simulink model "gyro"  (R2020a)
settings: Solver=daessc  StartTime=0.0  StopTime=0.35  RelTol=1e-3
values from neighbouring files (symbols this model uses):
  m = 0.5    [init_2021_03_10.m]
  ts = 1e-4    (= 0.0001)    [init_2021_03_10.m]
libraries: fl_lib x33, nesl_utility x8
settings Model: Creator=dbagn  LastModifiedBy=dbagn

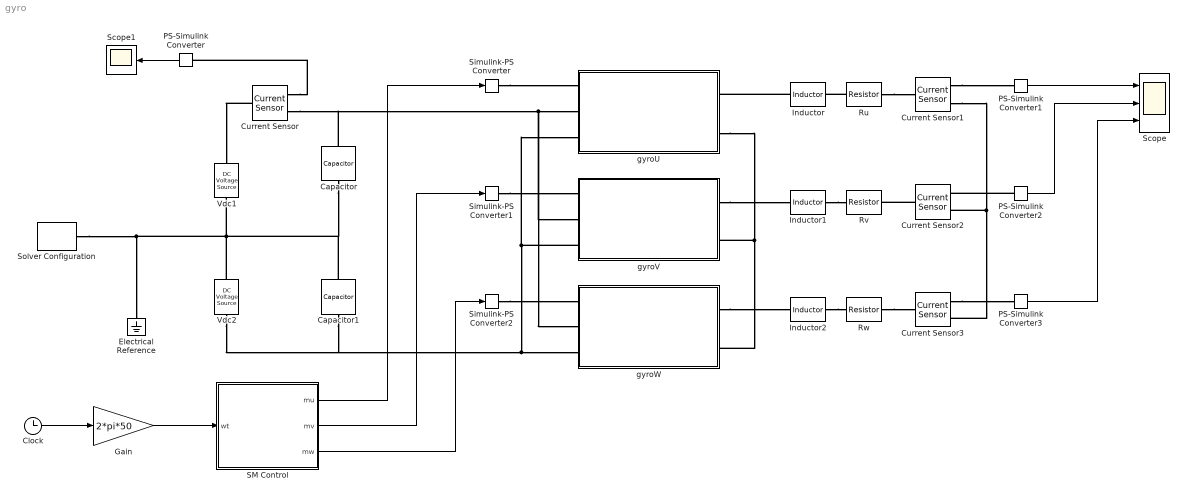
== system gyro ==
  Capacitor : fl_lib/Electrical/Electrical Elements/Capacitor  c=5e-3 F  r=1e-3 Ohm  g=0 1/Ohm  i_specify=off  i_priority=None  i=0 A  i_nominal_specify=off  i_nominal_unit=A  i_nominal_value=1  v_specify=off  v_priority=High  v=350 V  v_nominal_specify=off  v_nominal_unit=V  v_nominal_value=1  vc_specify=on  vc_priority=High  vc=350 V  vc_nominal_specify=off  vc_nominal_unit=V  vc_nominal_value=1
  Capacitor1 : fl_lib/Electrical/Electrical Elements/Capacitor  c=5e-3 F  r=1e-3 Ohm  g=0 1/Ohm  i_specify=off  i_priority=None  i=0 A  i_nominal_specify=off  i_nominal_unit=A  i_nominal_value=1  v_specify=off  v_priority=High  v=0 V  v_nominal_specify=off  v_nominal_unit=V  v_nominal_value=1  vc_specify=on  vc_priority=High  vc=350 V  vc_nominal_specify=off  vc_nominal_unit=V  vc_nominal_value=1
  Clock : Clock
  Current Sensor{,1..3} (4 alike) : fl_lib/Electrical/Electrical Sensors/Current Sensor
  Electrical Reference : fl_lib/Electrical/Electrical Elements/Electrical Reference
  Gain : Gain  Gain=2*pi*50
  Inductor : fl_lib/Electrical/Electrical Elements/Inductor  l=1e-4 H  r=0 Ohm  g=1e-9 1/Ohm  i_specify=off  i_priority=None  i=0 A  i_nominal_specify=off  i_nominal_unit=A  i_nominal_value=1  v_specify=off  v_priority=None  v=0 V  v_nominal_specify=off  v_nominal_unit=V  v_nominal_value=1  i_L_specify=off  i_L_priority=High  i_L=0 A  i_L_nominal_specify=off  i_L_nominal_unit=A  i_L_nominal_value=1
  Inductor1 : fl_lib/Electrical/Electrical Elements/Inductor  l=1e-4 H  r=0 Ohm  g=1e-9 1/Ohm  i_specify=off  i_priority=None  i=0 A  i_nominal_specify=off  i_nominal_unit=A  i_nominal_value=1  v_specify=off  v_priority=None  v=0 V  v_nominal_specify=off  v_nominal_unit=V  v_nominal_value=1  i_L_specify=off  i_L_priority=High  i_L=0 A  i_L_nominal_specify=off  i_L_nominal_unit=A  i_L_nominal_value=1
  Inductor2 : fl_lib/Electrical/Electrical Elements/Inductor  l=1e-4 H  r=0 Ohm  g=1e-9 1/Ohm  i_specify=off  i_priority=None  i=0 A  i_nominal_specify=off  i_nominal_unit=A  i_nominal_value=1  v_specify=off  v_priority=None  v=0 V  v_nominal_specify=off  v_nominal_unit=V  v_nominal_value=1  i_L_specify=off  i_L_priority=High  i_L=0 A  i_L_nominal_specify=off  i_L_nominal_unit=A  i_L_nominal_value=1
  PS-Simulink Converter{,1..3} (4 alike) : nesl_utility/PS-Simulink Converter  PhysicalDomain=network_engine_domain  SubClassName=ps_output  LeftPortType=input  RightPortType=output  PseudoPeriodic=off  Frequencies=[]  Unit=inherit  AffineConversion=off
  Ru : fl_lib/Electrical/Electrical Elements/Resistor  R=20 Ohm  i_specify=off  i_priority=None  i=0 A  i_nominal_specify=off  i_nominal_unit=A  i_nominal_value=1  v_specify=off  v_priority=None  v=0 V  v_nominal_specify=off  v_nominal_unit=V  v_nominal_value=1
  Rv : fl_lib/Electrical/Electrical Elements/Resistor  R=20 Ohm  i_specify=off  i_priority=None  i=0 A  i_nominal_specify=off  i_nominal_unit=A  i_nominal_value=1  v_specify=off  v_priority=None  v=0 V  v_nominal_specify=off  v_nominal_unit=V  v_nominal_value=1
  Rw : fl_lib/Electrical/Electrical Elements/Resistor  R=20 Ohm  i_specify=off  i_priority=None  i=0 A  i_nominal_specify=off  i_nominal_unit=A  i_nominal_value=1  v_specify=off  v_priority=None  v=0 V  v_nominal_specify=off  v_nominal_unit=V  v_nominal_value=1
  SM Control : Subsystem
  Scope : Scope  NumInputPorts=3
  Scope1 : Scope
  Simulink-PS Converter : nesl_utility/Simulink-PS Converter  PhysicalDomain=network_engine_domain  SubClassName=ps_input  LeftPortType=input  RightPortType=output  PseudoPeriodic=off  Frequencies=[]  NoiseDistribution=none  NoiseParameters=[]  Unit=1  AffineConversion=off  FilteringAndDerivatives=provide  SimscapeFilterOrder=1  InputFilterTimeConstant=0.001  UdotUserProvided=0
  Simulink-PS Converter1 : nesl_utility/Simulink-PS Converter  PhysicalDomain=network_engine_domain  SubClassName=ps_input  LeftPortType=input  RightPortType=output  PseudoPeriodic=off  Frequencies=[]  NoiseDistribution=none  NoiseParameters=[]  Unit=1  AffineConversion=off  FilteringAndDerivatives=provide  SimscapeFilterOrder=1  InputFilterTimeConstant=0.001  UdotUserProvided=0
  Simulink-PS Converter2 : nesl_utility/Simulink-PS Converter  PhysicalDomain=network_engine_domain  SubClassName=ps_input  LeftPortType=input  RightPortType=output  PseudoPeriodic=off  Frequencies=[]  NoiseDistribution=none  NoiseParameters=[]  Unit=1  AffineConversion=off  FilteringAndDerivatives=provide  SimscapeFilterOrder=1  InputFilterTimeConstant=0.001  UdotUserProvided=0
  Solver Configuration : nesl_utility/Solver Configuration  PhysicalDomain=network_engine_domain  SubClassName=solver  LeftPortType=input  RightPortType=generic  Tones=[]  Harmonics=[]  SimulateNoise=off  Profile=off  UseLocalSampling=off  EnableSwitchedLinearOptims=on  FrequencyDomain=off  UseCCode=off  RelTol=0.001  AbsTol=1e-06  MinStep=1e-09  ToWorkspace=off  RevertToSquareIcSolve=off  NumHomotopyIterations=100  PhasorMode=off  PhasorModeNumHarmonics=1  DoDC=off  ResidualTolerance=1e-09  UseLocalSolver=on  LocalSolverChoice=NE_BACKWARD_EULER_ADVANCER  LocalSolverSampleTime=ts  DoFixedCost=on  MaxNonlinIter=3  MaxModeIter=2  LinearAlgebra=auto  EquationFormulation=NE_TIME_EF  DelaysMemoryBudget=1024  AutomaticFiltering=on  FilteringTimeConstant=0.001  PartitionStorageMethod=AS_NEEDED  PartitionMemoryBudget=1024  PartitionMethod=ROBUST
  Vdc1 : fl_lib/Electrical/Electrical Sources/DC Voltage Source  v0=350 V
  Vdc2 : fl_lib/Electrical/Electrical Sources/DC Voltage Source  v0=350 V
  gyroU : Subsystem
  gyroV : Subsystem
  gyroW : Subsystem
  wires:
  Clock/1 -> Gain/1
  Gain/1 -> SM Control/1(wt)
  SM Control/1(mu) -> Simulink-PS Converter/1
  SM Control/2(mv) -> Simulink-PS Converter1/1
  SM Control/3(mw) -> Simulink-PS Converter2/1
  PS-Simulink Converter1/1 -> Scope/1
  PS-Simulink Converter2/1 -> Scope/2
  PS-Simulink Converter3/1 -> Scope/3
  PS-Simulink Converter/1 -> Scope1/1
  connections:
  gyroW/LConn2 -- gyroV/LConn2 -- Capacitor/LConn1 -- Current Sensor/RConn2 -- gyroU/LConn2
  Vdc2/LConn1 -- Capacitor1/LConn1 -- Capacitor/RConn1 -- Solver Configuration/RConn1 -- Electrical Reference/LConn1 -- Vdc1/RConn1
  gyroV/LConn3 -- Capacitor1/RConn1 -- Vdc2/RConn1 -- gyroW/LConn3 -- gyroU/LConn3
  gyroU/RConn2 -- gyroW/RConn2 -- gyroV/RConn2
  Ru/LConn1 -- Inductor/RConn1
  Inductor1/RConn1 -- Rv/LConn1
  gyroW/RConn1 -- Inductor2/LConn1
  Simulink-PS Converter/RConn1 -- gyroU/LConn1
  Simulink-PS Converter1/RConn1 -- gyroV/LConn1
  Simulink-PS Converter2/RConn1 -- gyroW/LConn1
  Current Sensor/LConn1 -- Vdc1/LConn1
  Current Sensor/RConn1 -- PS-Simulink Converter/LConn1
  Ru/RConn1 -- Current Sensor1/LConn1
  Current Sensor2/LConn1 -- Rv/RConn1
  Rw/RConn1 -- Current Sensor3/LConn1
  Current Sensor1/RConn2 -- Current Sensor3/RConn2 -- Current Sensor2/RConn2
  Current Sensor1/RConn1 -- PS-Simulink Converter1/LConn1
  PS-Simulink Converter2/LConn1 -- Current Sensor2/RConn1
  Current Sensor3/RConn1 -- PS-Simulink Converter3/LConn1
  Inductor/LConn1 -- gyroU/RConn1
  gyroV/RConn1 -- Inductor1/LConn1
  Inductor2/RConn1 -- Rw/LConn1

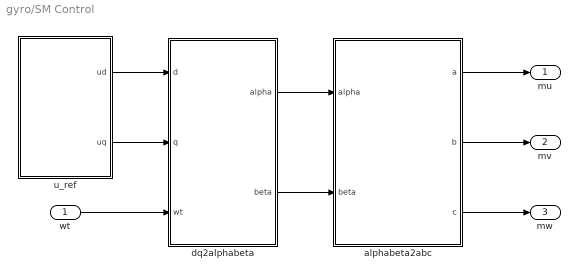
== system gyro/SM Control ==
  wt : Inport
  alphabeta2abc : Subsystem
  dq2alphabeta : Subsystem
  u_ref : Subsystem
  mu : Outport  VectorParamsAs1DForOutWhenUnconnected=off
  mv : Outport  Port=2  VectorParamsAs1DForOutWhenUnconnected=off
  mw : Outport  Port=3  VectorParamsAs1DForOutWhenUnconnected=off
  wires:
  wt/1 -> dq2alphabeta/3(wt)
  u_ref/2(uq) -> dq2alphabeta/2(q)
  u_ref/1(ud) -> dq2alphabeta/1(d)
  dq2alphabeta/2(beta) -> alphabeta2abc/2(beta)
  dq2alphabeta/1(alpha) -> alphabeta2abc/1(alpha)
  alphabeta2abc/1(a) -> mu/1
  alphabeta2abc/2(b) -> mv/1
  alphabeta2abc/3(c) -> mw/1

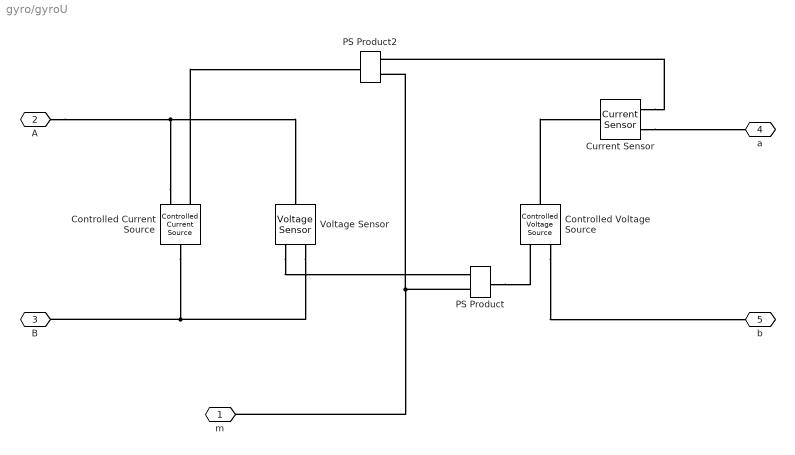
== system gyro/gyroU ==
  Controlled Current Source : fl_lib/Electrical/Electrical Sources/Controlled Current Source
  Controlled Voltage Source : fl_lib/Electrical/Electrical Sources/Controlled Voltage Source
  Current Sensor : fl_lib/Electrical/Electrical Sensors/Current Sensor
  PS Product : fl_lib/Physical Signals/Functions/PS Product
  PS Product2 : fl_lib/Physical Signals/Functions/PS Product
  Voltage Sensor : fl_lib/Electrical/Electrical Sensors/Voltage Sensor
  m : PMIOPort  Side=Left
  A : PMIOPort  Port=2  Side=Left
  B : PMIOPort  Port=3  Side=Left
  a : PMIOPort  Port=4  Side=Right
  b : PMIOPort  Port=5  Side=Right
  connections:
  Controlled Voltage Source/LConn1 -- Current Sensor/LConn1
  Controlled Voltage Source/RConn2 -- b/RConn1
  Controlled Current Source/RConn1 -- PS Product2/RConn1
  Controlled Current Source/RConn2 -- A/RConn1 -- Voltage Sensor/LConn1
  PS Product/LConn2 -- PS Product2/LConn1 -- m/RConn1
  Controlled Current Source/LConn1 -- B/RConn1 -- Voltage Sensor/RConn2
  Current Sensor/RConn2 -- a/RConn1
  PS Product/RConn1 -- Controlled Voltage Source/RConn1
  Voltage Sensor/RConn1 -- PS Product/LConn1
  Current Sensor/RConn1 -- PS Product2/LConn2

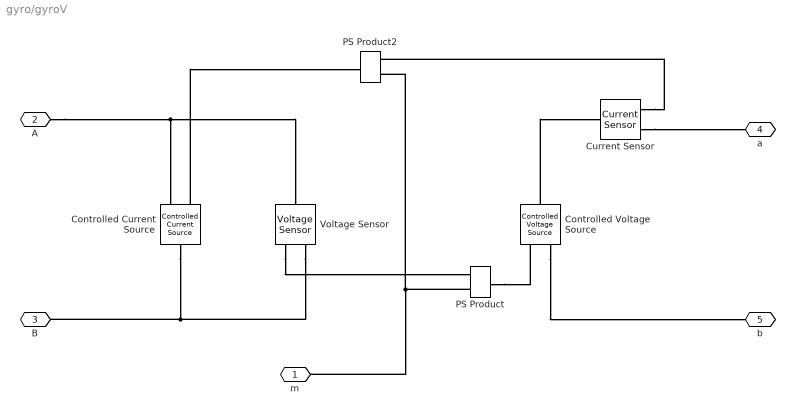
== system gyro/gyroV ==
  Controlled Current Source : fl_lib/Electrical/Electrical Sources/Controlled Current Source
  Controlled Voltage Source : fl_lib/Electrical/Electrical Sources/Controlled Voltage Source
  Current Sensor : fl_lib/Electrical/Electrical Sensors/Current Sensor
  PS Product : fl_lib/Physical Signals/Functions/PS Product
  PS Product2 : fl_lib/Physical Signals/Functions/PS Product
  Voltage Sensor : fl_lib/Electrical/Electrical Sensors/Voltage Sensor
  m : PMIOPort  Side=Left
  A : PMIOPort  Port=2  Side=Left
  B : PMIOPort  Port=3  Side=Left
  a : PMIOPort  Port=4  Side=Right
  b : PMIOPort  Port=5  Side=Right
  connections:
  Current Sensor/RConn1 -- PS Product2/LConn2
  Voltage Sensor/RConn1 -- PS Product/LConn1
  PS Product/RConn1 -- Controlled Voltage Source/RConn1
  Current Sensor/RConn2 -- a/RConn1
  B/RConn1 -- Controlled Current Source/LConn1 -- Voltage Sensor/RConn2
  PS Product2/LConn1 -- PS Product/LConn2 -- m/RConn1
  A/RConn1 -- Controlled Current Source/RConn2 -- Voltage Sensor/LConn1
  Controlled Current Source/RConn1 -- PS Product2/RConn1
  Controlled Voltage Source/RConn2 -- b/RConn1
  Controlled Voltage Source/LConn1 -- Current Sensor/LConn1

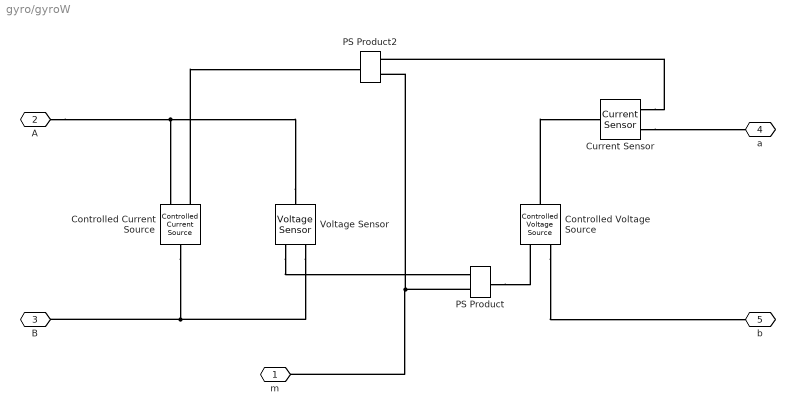
== system gyro/gyroW ==
  Controlled Current Source : fl_lib/Electrical/Electrical Sources/Controlled Current Source
  Controlled Voltage Source : fl_lib/Electrical/Electrical Sources/Controlled Voltage Source
  Current Sensor : fl_lib/Electrical/Electrical Sensors/Current Sensor
  PS Product : fl_lib/Physical Signals/Functions/PS Product
  PS Product2 : fl_lib/Physical Signals/Functions/PS Product
  Voltage Sensor : fl_lib/Electrical/Electrical Sensors/Voltage Sensor
  m : PMIOPort  Side=Left
  A : PMIOPort  Port=2  Side=Left
  B : PMIOPort  Port=3  Side=Left
  a : PMIOPort  Port=4  Side=Right
  b : PMIOPort  Port=5  Side=Right
  connections:
  Controlled Voltage Source/LConn1 -- Current Sensor/LConn1
  Controlled Voltage Source/RConn2 -- b/RConn1
  Controlled Current Source/RConn1 -- PS Product2/RConn1
  Voltage Sensor/LConn1 -- Controlled Current Source/RConn2 -- A/RConn1
  m/RConn1 -- PS Product/LConn2 -- PS Product2/LConn1
  Voltage Sensor/RConn2 -- Controlled Current Source/LConn1 -- B/RConn1
  Current Sensor/RConn2 -- a/RConn1
  PS Product/RConn1 -- Controlled Voltage Source/RConn1
  Voltage Sensor/RConn1 -- PS Product/LConn1
  Current Sensor/RConn1 -- PS Product2/LConn2

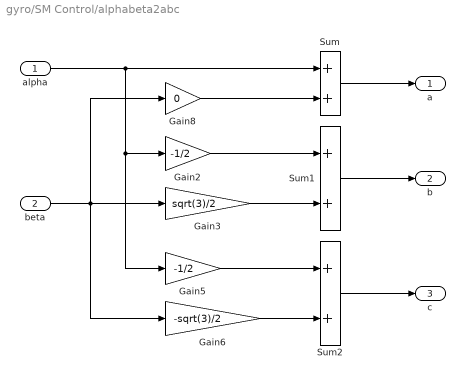
== system gyro/SM Control/alphabeta2abc ==
  alpha : Inport
  beta : Inport  Port=2
  Gain2 : Gain  Gain=-1/2
  Gain3 : Gain  Gain=sqrt(3)/2
  Gain5 : Gain  Gain=-1/2
  Gain6 : Gain  Gain=-sqrt(3)/2
  Gain8 : Gain  Gain=0
  Sum : Sum
  Sum1 : Sum
  Sum2 : Sum
  a : Outport  VectorParamsAs1DForOutWhenUnconnected=off
  b : Outport  Port=2  VectorParamsAs1DForOutWhenUnconnected=off
  c : Outport  Port=3  VectorParamsAs1DForOutWhenUnconnected=off
  wires:
  Gain2/1 -> Sum1/1
  Gain3/1 -> Sum1/2
  Gain5/1 -> Sum2/1
  Gain6/1 -> Sum2/2
  alpha/1 -> Sum/1, Gain2/1, Gain5/1
  beta/1 -> Gain3/1, Gain6/1, Gain8/1
  Sum/1 -> a/1
  Sum1/1 -> b/1
  Sum2/1 -> c/1
  Gain8/1 -> Sum/2

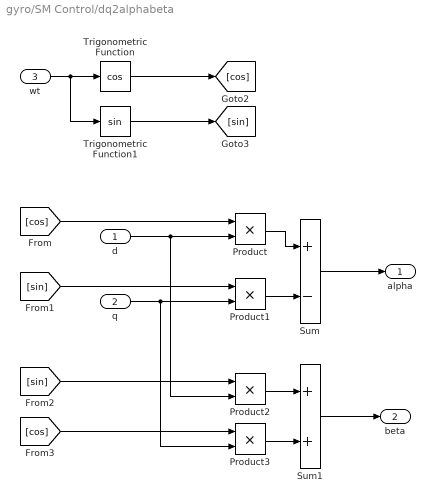
== system gyro/SM Control/dq2alphabeta ==
  d : Inport
  q : Inport  Port=2
  wt : Inport  Port=3
  Product{,1..3} (4 alike) : Product  RndMeth=Zero
  Sum : Sum  Inputs=+-
  Sum1 : Sum
  Trigonometric Function : Trigonometry  Operator=cos
  Trigonometric Function1 : Trigonometry
  alpha : Outport  VectorParamsAs1DForOutWhenUnconnected=off
  beta : Outport  Port=2  VectorParamsAs1DForOutWhenUnconnected=off
  wires:
  Sum1/1 -> beta/1
  [cos] -> Product3/1
  Product3/1 -> Sum1/2
  Product2/1 -> Sum1/1
  [sin] -> Product2/1
  Sum/1 -> alpha/1
  q/1 -> Product3/2, Product1/2
  [sin] -> Product1/1
  Product1/1 -> Sum/2
  Product/1 -> Sum/1
  d/1 -> Product2/2, Product/2
  [cos] -> Product/1
  Trigonometric Function1/1 -> [sin]
  Trigonometric Function/1 -> [cos]
  wt/1 -> Trigonometric Function/1, Trigonometric Function1/1

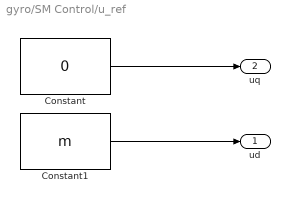
== system gyro/SM Control/u_ref ==
  Constant : Constant  Value=0  SampleTime=ts
  Constant1 : Constant  Value=m  SampleTime=ts
  ud : Outport  VectorParamsAs1DForOutWhenUnconnected=off
  uq : Outport  Port=2  VectorParamsAs1DForOutWhenUnconnected=off
  wires:
  Constant/1 -> uq/1
  Constant1/1 -> ud/1
